simulink model "nonlinear2"  (R2016a)
settings: Solver=ode8  StartTime=0.0  StopTime=Ts  FixedStep=sampletime  RelTol=1e-3
values from neighbouring files (symbols this model uses):
  S1 = S(end)    [MACm.m]
  T_g1 = T_g(end)    [MACm.m]
  Teta1 = Teta(end)    [MACm.m]
  u1 = 11.9    [MACm.m]    (also in Test.m = U1(1,i))
  u11 = U1(1,i)    [MACm.m]
  u2 = 2130    [MACm.m]    (also in Test.m = U2(1,i))
  u22 = U2(1,i)    [MACm.m]
  w_g1 = w_g(end)    [MACm.m]
  w_r1 = w_r(end)    [MACm.m]
settings Model: Creator=mrutn  LastModifiedBy=mrutn

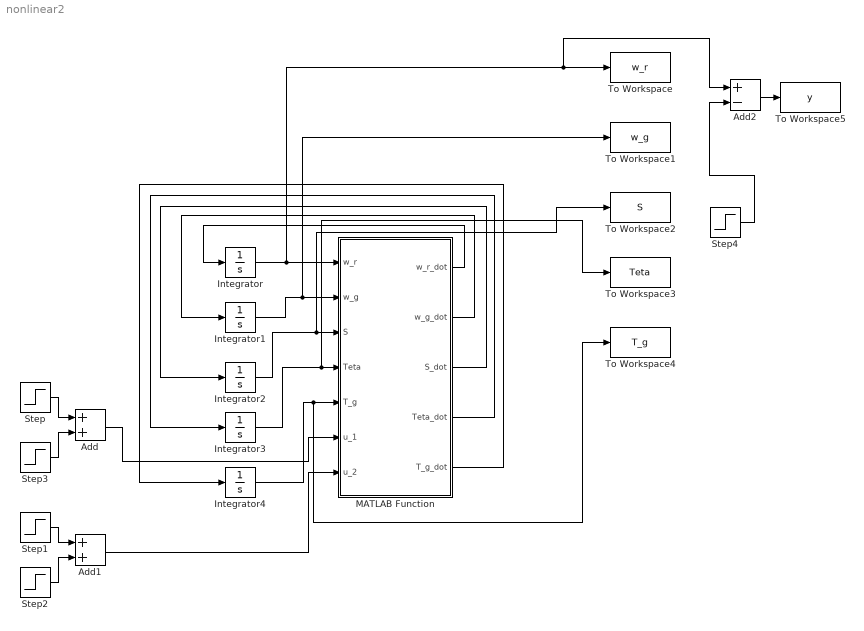
== system nonlinear2 ==
  Add : Sum
  Add1 : Sum
  Add2 : Sum  Inputs=+-
  Integrator : Integrator  InitialCondition=w_r1
  Integrator1 : Integrator  InitialCondition=w_g1
  Integrator2 : Integrator  InitialCondition=S1
  Integrator3 : Integrator  InitialCondition=Teta1
  Integrator4 : Integrator  InitialCondition=T_g1
  MATLAB Function : MATLAB Function  TreatAsAtomicUnit=on
  Step : Step  Time=0  After=u1  SampleTime=0
  Step1 : Step  Time=0  After=u2  SampleTime=0
  Step2 : Step  Time=0  After=u22  SampleTime=0
  Step3 : Step  Time=0  After=u11  SampleTime=0
  Step4 : Step  Time=0  After=0.072676784965328  SampleTime=0
  To Workspace : ToWorkspace  VariableName=w_r  SampleTime=-1
  To Workspace1 : ToWorkspace  VariableName=w_g  SampleTime=-1
  To Workspace2 : ToWorkspace  VariableName=S  SampleTime=-1
  To Workspace3 : ToWorkspace  VariableName=Teta  SampleTime=-1
  To Workspace4 : ToWorkspace  VariableName=T_g  SampleTime=-1
  To Workspace5 : ToWorkspace  VariableName=y  SampleTime=-1
  wires:
  Integrator/1 -> Add2/1, To Workspace/1, MATLAB Function/1(w_r)
  MATLAB Function/4(Teta_dot) -> Integrator3/1
  MATLAB Function/5(T_g_dot) -> Integrator4/1
  Integrator4/1 -> To Workspace4/1, MATLAB Function/5(T_g)
  MATLAB Function/1(w_r_dot) -> Integrator/1
  MATLAB Function/3(S_dot) -> Integrator2/1
  Integrator2/1 -> To Workspace2/1, MATLAB Function/3(S)
  Integrator3/1 -> To Workspace3/1, MATLAB Function/4(Teta)
  MATLAB Function/2(w_g_dot) -> Integrator1/1
  Integrator1/1 -> To Workspace1/1, MATLAB Function/2(w_g)
  Step/1 -> Add/1
  Step3/1 -> Add/2
  Step1/1 -> Add1/1
  Step2/1 -> Add1/2
  Add1/1 -> MATLAB Function/7(u_2)
  Add/1 -> MATLAB Function/6(u_1)
  Add2/1 -> To Workspace5/1
  Step4/1 -> Add2/2

== matlab function nonlinear2/MATLAB Function ==
  data: w_r input; w_r_dot output; w_g input; S input; Teta input; T_g input; u_1 input; u_2 input; w_g_dot output; S_dot output; Teta_dot output; T_g_dot output
function [w_r_dot ,w_g_dot ,S_dot ,Teta_dot ,T_g_dot] = fcn(w_r,w_g,S,Teta,T_g,u_1,u_2)
%#codegen
Ds=8e+4;
Jr=90000;
Ng=24.6;
Ks=8e+6;
Jg=10;
Tou_teta=0.15;
Tou_T=0.1;
Rou=1.2;
R=14.5;
v=14;

Landa=(v/R)/w_r;
Landa_t_inv=(1/(inv(Landa)+0.12*Teta))-(0.035/((1.5*Teta)^3+1));
C_p=0.22*((116*Landa_t_inv)-0.6*Teta-5)*exp(-12.5*Landa_t_inv);
P_r=0.5*Rou*pi*(R^2)*(v^3)*C_p;

w_r_dot=(P_r/(Jr*w_r))-((Ds*w_r)/Jr)+((Ds*w_g)/(Jr*Ng))-((Ks*S)/Jr);
w_g_dot=((Ds*w_r)/(Jg*Ng))-((Ds*w_g)/(Jg*Ng*Ng))+((Ks*S)/(Jg*Ng))-(T_g/Jg);
S_dot=w_r-(w_g/Ng);
Teta_dot=-(Teta/Tou_teta)+(u_1/Tou_teta);
T_g_dot=-(T_g/Tou_T)+(u_2/Tou_T);
